simulink model "ekf_2d"  (R2024b)
settings: Solver=ode1  StartTime=0.0  StopTime=30  FixedStep=0.1  RelTol=1e-3
settings Model: Creator=rasim  LastModifiedBy=rasim

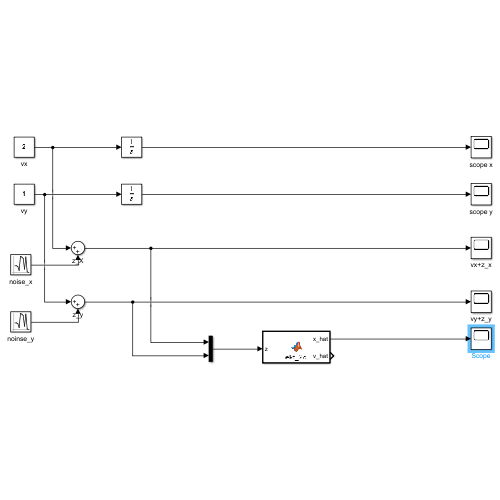
[thumbnail: Simulink's stored preview of the top-level diagram]
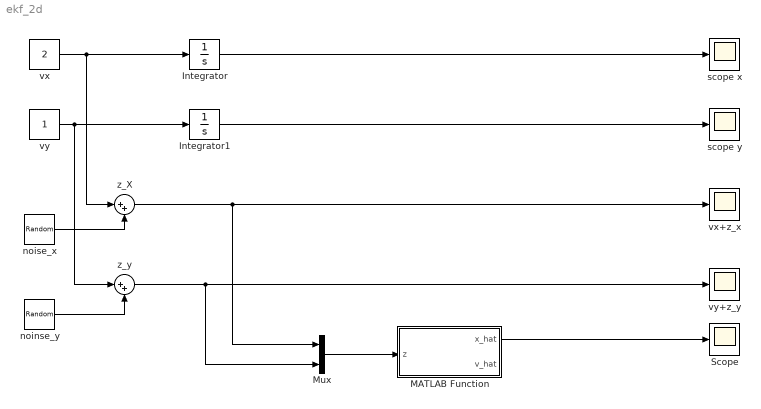
== system ekf_2d ==
  Integrator : Integrator
  Integrator1 : Integrator
  MATLAB Function : MATLAB Function  TreatAsAtomicUnit=on
  Mux : Mux  Inputs=2
  Scope : Scope
  "noinse_y " : RandomNumber  SampleTime=0.1
  "noise_x " : RandomNumber  SampleTime=0.1
  scope x : Scope
  scope y : Scope
  vx : Constant  Value=2
  vx+z_x : Scope
  vy : Constant
  vy+z_y : Scope
  z_X : Sum  Inputs=|++
  z_y : Sum  Inputs=|++
  wires:
  vx/1 -> z_X/1, Integrator/1
  vy/1 -> z_y/1, Integrator1/1
  Integrator/1 -> scope x/1
  Integrator1/1 -> scope y/1
  "noise_x "/1 -> z_X/2
  "noinse_y "/1 -> z_y/2
  z_X/1 -> Mux/1, vx+z_x/1
  z_y/1 -> Mux/2, vy+z_y/1
  MATLAB Function/1(x_hat) -> Scope/1
  Mux/1 -> MATLAB Function/1(z)

== matlab function ekf_2d/MATLAB Function ==
  data: z input; x_hat output; v_hat output
function [x_hat, v_hat] = ekf_2d(z)
    % z = [z_x; z_y]

    % Kalıcı değişkenler
    persistent x P dt
    if isempty(x)
        x = zeros(4,1);   % Başlangıç tahmini [x; y; vx; vy]
        P = eye(4);       % Kovaryans matrisi
        dt = 1;           % Zaman adımı
    end

    % Durum geçiş matrisi
    F = [1 0 dt 0;
         0 1 0 dt;
         0 0 1  0;
         0 0 0  1];

    % Ölçüm matrisi
    H = [1 0 0 0;
         0 1 0 0];

    % Gürültü kovaryansları
    Q = 0.01 * eye(4);   % Sistem gürültüsü
    R = 0.5  * eye(2);   % Ölçüm gürültüsü

    % 1. Öngörü (Prediction)
    x = F * x;
    P = F * P * F' + Q;

    % 2. Güncelleme (Measurement update)
    K = P * H' / (H * P * H' + R);  % Kalman kazancı
    x = x + K * (z - H * x);
    P = (eye(4) - K * H) * P;

    % Çıkışlar
    x_hat = x(1:2);  % Tahmini konum [x; y]
    v_hat = x(3:4);  % Tahmini hız [vx; vy]
end
